simulink library "MCI_lib"  (Simulink 7.5)
settings: Solver=ode45  StartTime=0.0  StopTime=10.0  RelTol=1e-3
values from neighbouring files (symbols this model uses):
  pMCI_bool_MotCtrlTqLimEna_C = Simulink.Parameter    [MCI_par.m]
  pMCI_m_TireDiam_C = Simulink.Parameter    [MCI_par.m]
  pMCI_Nm_DrvTqLim_C = Simulink.Parameter    [MCI_par.m]
  pMCI_Nm_RcpTqLim_C = Simulink.Parameter    [MCI_par.m]
  pMCI_ratio_DrvEff_MAP = Simulink.Parameter    [MCI_par.m]
  pMCI_ratio_KmPerHrToMtrPerSec_C = Simulink.Parameter    [MCI_par.m]
  pMCI_ratio_TrsmRat_C = Simulink.Parameter    [MCI_par.m]
  pMCI_rpm_InsteadVld_C = Simulink.Parameter    [MCI_par.m]
  pMCI_s_NoOfSec_C = Simulink.Parameter    [MCI_par.m]
undefined symbols (not defined in the file or in its folder): MotCtrlWrkStsTyp, p_bool_False_M, p_bool_True_M, p_st_DrvModeFlg_C
libraries: BaseOperationLib_Browser x79, PES_CZ_FAW x6, simulink x1
(part 1 of 2)
settings Model: Creator=wuaibin  LastModifiedBy=wuaibin

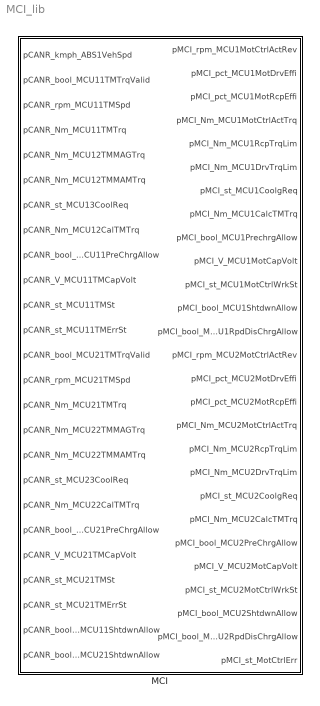
== system MCI_lib ==
  MCI : Subsystem  TreatAsAtomicUnit=on

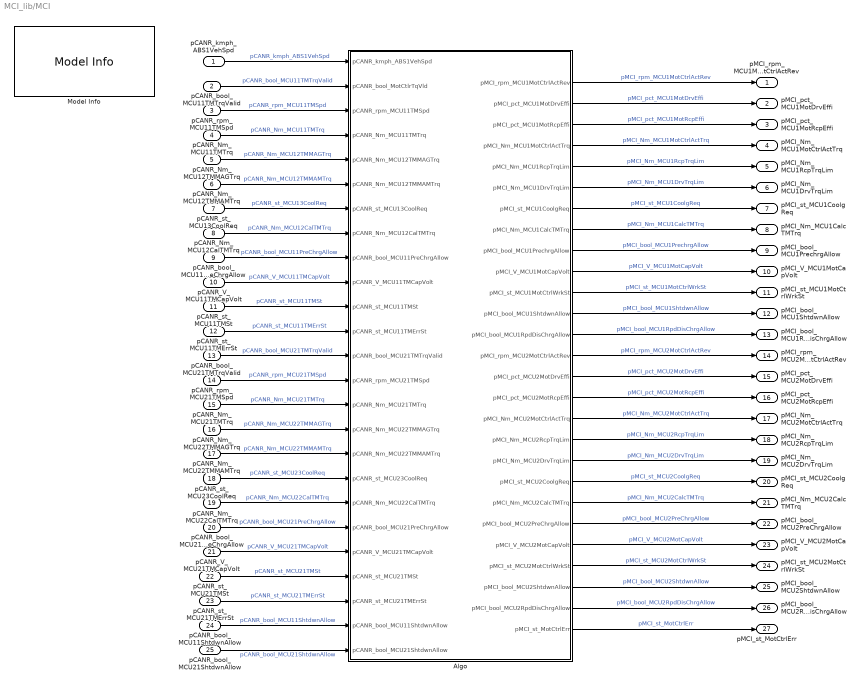
== system MCI_lib/MCI ==
  pCANR_kmph_ABS1VehSpd : Inport  OutDataType=fixdt(1, 16)  OutScaling=2^0
  pCANR_bool_MCU11TMTrqValid : Inport  Port=2
  pCANR_rpm_MCU11TMSpd : Inport  Port=3
  pCANR_Nm_MCU11TMTrq : Inport  Port=4
  pCANR_Nm_MCU12TMMAGTrq : Inport  Port=5
  pCANR_Nm_MCU12TMMAMTrq : Inport  Port=6
  pCANR_st_MCU13CoolReq : Inport  Port=7  OutDataType=fixdt(1, 16)  OutScaling=2^0
  pCANR_Nm_MCU12CalTMTrq : Inport  Port=8  OutDataType=fixdt(1, 16)  OutScaling=2^0
  pCANR_bool_MCU11PreChrgAllow : Inport  Port=9  OutDataType=fixdt(1, 16)  OutScaling=2^0
  pCANR_V_MCU11TMCapVolt : Inport  Port=10  OutDataType=fixdt(1, 16)  OutScaling=2^0
  pCANR_st_MCU11TMSt : Inport  Port=11  OutDataType=fixdt(1, 16)  OutScaling=2^0
  pCANR_st_MCU11TMErrSt : Inport  Port=12  OutDataType=fixdt(1, 16)  OutScaling=2^0
  pCANR_bool_MCU21TMTrqValid : Inport  Port=13
  pCANR_rpm_MCU21TMSpd : Inport  Port=14
  pCANR_Nm_MCU21TMTrq : Inport  Port=15
  pCANR_Nm_MCU22TMMAGTrq : Inport  Port=16  OutDataType=fixdt(1, 16)  OutScaling=2^0
  pCANR_Nm_MCU22TMMAMTrq : Inport  Port=17
  pCANR_st_MCU23CoolReq : Inport  Port=18  OutDataType=fixdt(1, 16)  OutScaling=2^0
  pCANR_Nm_MCU22CalTMTrq : Inport  Port=19  OutDataType=fixdt(1, 16)  OutScaling=2^0
  pCANR_bool_MCU21PreChrgAllow : Inport  Port=20
  pCANR_V_MCU21TMCapVolt : Inport  Port=21
  pCANR_st_MCU21TMSt : Inport  Port=22  OutDataType=fixdt(1, 16)  OutScaling=2^0
  pCANR_st_MCU21TMErrSt : Inport  Port=23  OutDataType=fixdt(1, 16)  OutScaling=2^0
  pCANR_bool_MCU11ShtdwnAllow : Inport  Port=24  OutDataType=fixdt(1, 16)  OutScaling=2^0
  pCANR_bool_MCU21ShtdwnAllow : Inport  Port=25  OutDataType=fixdt(1, 16)  OutScaling=2^0
  Algo : Subsystem
  Model Info : simulink/Model-Wide Utilities/Model Info  SystemSampleTime=-1  InitialBlockCM=None  BlockCM=None  Frame=on  DisplayStringWithTags=Model Info\nCreated: %<Created>\nCreator: wuaibin  HorizontalTextAlignment=Center  LeftAlignmentValue=0.5  SourceBlockDiagram=HQEV_HCU  TagMaxNumber=20
  pMCI_rpm_MCU1MotCtrlActRev : Outport  OutDataType=fixdt(1, 16)  OutScaling=2^0
  pMCI_pct_MCU1MotDrvEffi : Outport  Port=2  OutDataType=fixdt(1, 16)  OutScaling=2^0
  pMCI_pct_MCU1MotRcpEffi : Outport  Port=3  OutDataType=fixdt(1, 16)  OutScaling=2^0
  pMCI_Nm_MCU1MotCtrlActTrq : Outport  Port=4  OutDataType=fixdt(1, 16)  OutScaling=2^0
  pMCI_Nm_MCU1RcpTrqLim : Outport  Port=5  OutDataType=fixdt(1, 16)  OutScaling=2^0
  pMCI_Nm_MCU1DrvTrqLim : Outport  Port=6  OutDataType=fixdt(1, 16)  OutScaling=2^0
  pMCI_st_MCU1CoolgReq : Outport  Port=7  OutDataType=fixdt(1, 16)  OutScaling=2^0
  pMCI_Nm_MCU1CalcTMTrq : Outport  Port=8  OutDataType=fixdt(1, 16)  OutScaling=2^0
  pMCI_bool_MCU1PrechrgAllow : Outport  Port=9  OutDataType=fixdt(1, 16)  OutScaling=2^0
  pMCI_V_MCU1MotCapVolt : Outport  Port=10  OutDataType=fixdt(1, 16)  OutScaling=2^0
  pMCI_st_MCU1MotCtrlWrkSt : Outport  Port=11  OutDataType=fixdt(1, 16)  OutScaling=2^0
  pMCI_bool_MCU1ShtdwnAllow : Outport  Port=12  OutDataType=fixdt(1, 16)  OutScaling=2^0
  pMCI_bool_MCU1RpdDisChrgAllow : Outport  Port=13  OutDataType=fixdt(1, 16)  OutScaling=2^0
  pMCI_rpm_MCU2MotCtrlActRev : Outport  Port=14  OutDataType=fixdt(1, 16)  OutScaling=2^0
  pMCI_pct_MCU2MotDrvEffi : Outport  Port=15  OutDataType=fixdt(1, 16)  OutScaling=2^0
  pMCI_pct_MCU2MotRcpEffi : Outport  Port=16  OutDataType=fixdt(1, 16)  OutScaling=2^0
  pMCI_Nm_MCU2MotCtrlActTrq : Outport  Port=17  OutDataType=fixdt(1, 16)  OutScaling=2^0
  pMCI_Nm_MCU2RcpTrqLim : Outport  Port=18  OutDataType=fixdt(1, 16)  OutScaling=2^0
  pMCI_Nm_MCU2DrvTrqLim : Outport  Port=19  OutDataType=fixdt(1, 16)  OutScaling=2^0
  pMCI_st_MCU2CoolgReq : Outport  Port=20  OutDataType=fixdt(1, 16)  OutScaling=2^0
  pMCI_Nm_MCU2CalcTMTrq : Outport  Port=21  OutDataType=fixdt(1, 16)  OutScaling=2^0
  pMCI_bool_MCU2PreChrgAllow : Outport  Port=22  OutDataType=fixdt(1, 16)  OutScaling=2^0
  pMCI_V_MCU2MotCapVolt : Outport  Port=23  OutDataType=fixdt(1, 16)  OutScaling=2^0
  pMCI_st_MCU2MotCtrlWrkSt : Outport  Port=24  OutDataType=fixdt(1, 16)  OutScaling=2^0
  pMCI_bool_MCU2ShtdwnAllow : Outport  Port=25  OutDataType=fixdt(1, 16)  OutScaling=2^0
  pMCI_bool_MCU2RpdDisChrgAllow : Outport  Port=26  OutDataType=fixdt(1, 16)  OutScaling=2^0
  pMCI_st_MotCtrlErr : Outport  Port=27
  wires:
  pCANR_bool_MCU21TMTrqValid/1 -> Algo/13(pCANR_bool_MCU21TMTrqValid)  "pCANR_bool_MCU21TMTrqValid"
  pCANR_bool_MCU11TMTrqValid/1 -> Algo/2(pCANR_bool_MotCtlrTqVld)  "pCANR_bool_MCU11TMTrqValid"
  Algo/26(pMCI_bool_MCU2RpdDisChrgAllow) -> pMCI_bool_MCU2RpdDisChrgAllow/1  "pMCI_bool_MCU2RpdDisChrgAllow"
  Algo/13(pMCI_bool_MCU1RpdDisChrgAllow) -> pMCI_bool_MCU1RpdDisChrgAllow/1  "pMCI_bool_MCU1RpdDisChrgAllow"
  pCANR_st_MCU11TMErrSt/1 -> Algo/12(pCANR_st_MCU11TMErrSt)  "pCANR_st_MCU11TMErrSt"
  pCANR_st_MCU21TMErrSt/1 -> Algo/23(pCANR_st_MCU21TMErrSt)  "pCANR_st_MCU21TMErrSt"
  Algo/25(pMCI_bool_MCU2ShtdwnAllow) -> pMCI_bool_MCU2ShtdwnAllow/1  "pMCI_bool_MCU2ShtdwnAllow"
  Algo/12(pMCI_bool_MCU1ShtdwnAllow) -> pMCI_bool_MCU1ShtdwnAllow/1  "pMCI_bool_MCU1ShtdwnAllow"
  Algo/27(pMCI_st_MotCtrlErr) -> pMCI_st_MotCtrlErr/1  "pMCI_st_MotCtrlErr"
  pCANR_st_MCU21TMSt/1 -> Algo/22(pCANR_st_MCU21TMSt)  "pCANR_st_MCU21TMSt"
  pCANR_V_MCU21TMCapVolt/1 -> Algo/21(pCANR_V_MCU21TMCapVolt)  "pCANR_V_MCU21TMCapVolt"
  pCANR_bool_MCU21PreChrgAllow/1 -> Algo/20(pCANR_bool_MCU21PreChrgAllow)  "pCANR_bool_MCU21PreChrgAllow"
  pCANR_Nm_MCU22CalTMTrq/1 -> Algo/19(pCANR_Nm_MCU22CalTMTrq)  "pCANR_Nm_MCU22CalTMTrq"
  pCANR_st_MCU23CoolReq/1 -> Algo/18(pCANR_st_MCU23CoolReq)  "pCANR_st_MCU23CoolReq"
  pCANR_Nm_MCU22TMMAMTrq/1 -> Algo/17(pCANR_Nm_MCU22TMMAMTrq)  "pCANR_Nm_MCU22TMMAMTrq"
  pCANR_Nm_MCU22TMMAGTrq/1 -> Algo/16(pCANR_Nm_MCU22TMMAGTrq)  "pCANR_Nm_MCU22TMMAGTrq"
  pCANR_Nm_MCU21TMTrq/1 -> Algo/15(pCANR_Nm_MCU21TMTrq)  "pCANR_Nm_MCU21TMTrq"
  pCANR_rpm_MCU21TMSpd/1 -> Algo/14(pCANR_rpm_MCU21TMSpd)  "pCANR_rpm_MCU21TMSpd"
  Algo/1(pMCI_rpm_MCU1MotCtrlActRev) -> pMCI_rpm_MCU1MotCtrlActRev/1  "pMCI_rpm_MCU1MotCtrlActRev"
  pCANR_kmph_ABS1VehSpd/1 -> Algo/1(pCANR_kmph_ABS1VehSpd)  "pCANR_kmph_ABS1VehSpd"
  Algo/2(pMCI_pct_MCU1MotDrvEffi) -> pMCI_pct_MCU1MotDrvEffi/1  "pMCI_pct_MCU1MotDrvEffi"
  pCANR_rpm_MCU11TMSpd/1 -> Algo/3(pCANR_rpm_MCU11TMSpd)  "pCANR_rpm_MCU11TMSpd"
  Algo/3(pMCI_pct_MCU1MotRcpEffi) -> pMCI_pct_MCU1MotRcpEffi/1  "pMCI_pct_MCU1MotRcpEffi"
  pCANR_Nm_MCU11TMTrq/1 -> Algo/4(pCANR_Nm_MCU11TMTrq)  "pCANR_Nm_MCU11TMTrq"
  Algo/4(pMCI_Nm_MCU1MotCtrlActTrq) -> pMCI_Nm_MCU1MotCtrlActTrq/1  "pMCI_Nm_MCU1MotCtrlActTrq"
  pCANR_Nm_MCU12TMMAGTrq/1 -> Algo/5(pCANR_Nm_MCU12TMMAGTrq)  "pCANR_Nm_MCU12TMMAGTrq"
  Algo/5(pMCI_Nm_MCU1RcpTrqLim) -> pMCI_Nm_MCU1RcpTrqLim/1  "pMCI_Nm_MCU1RcpTrqLim"
  Algo/6(pMCI_Nm_MCU1DrvTrqLim) -> pMCI_Nm_MCU1DrvTrqLim/1  "pMCI_Nm_MCU1DrvTrqLim"
  pCANR_Nm_MCU12TMMAMTrq/1 -> Algo/6(pCANR_Nm_MCU12TMMAMTrq)  "pCANR_Nm_MCU12TMMAMTrq"
  Algo/7(pMCI_st_MCU1CoolgReq) -> pMCI_st_MCU1CoolgReq/1  "pMCI_st_MCU1CoolgReq"
  pCANR_st_MCU13CoolReq/1 -> Algo/7(pCANR_st_MCU13CoolReq)  "pCANR_st_MCU13CoolReq"
  Algo/8(pMCI_Nm_MCU1CalcTMTrq) -> pMCI_Nm_MCU1CalcTMTrq/1  "pMCI_Nm_MCU1CalcTMTrq"
  pCANR_Nm_MCU12CalTMTrq/1 -> Algo/8(pCANR_Nm_MCU12CalTMTrq)  "pCANR_Nm_MCU12CalTMTrq"
  pCANR_bool_MCU11PreChrgAllow/1 -> Algo/9(pCANR_bool_MCU11PreChrgAllow)  "pCANR_bool_MCU11PreChrgAllow"
  Algo/9(pMCI_bool_MCU1PrechrgAllow) -> pMCI_bool_MCU1PrechrgAllow/1  "pMCI_bool_MCU1PrechrgAllow"
  pCANR_V_MCU11TMCapVolt/1 -> Algo/10(pCANR_V_MCU11TMCapVolt)  "pCANR_V_MCU11TMCapVolt"
  pCANR_st_MCU11TMSt/1 -> Algo/11(pCANR_st_MCU11TMSt)  "pCANR_st_MCU11TMSt"
  Algo/10(pMCI_V_MCU1MotCapVolt) -> pMCI_V_MCU1MotCapVolt/1  "pMCI_V_MCU1MotCapVolt"
  Algo/11(pMCI_st_MCU1MotCtrlWrkSt) -> pMCI_st_MCU1MotCtrlWrkSt/1  "pMCI_st_MCU1MotCtrlWrkSt"
  Algo/14(pMCI_rpm_MCU2MotCtrlActRev) -> pMCI_rpm_MCU2MotCtrlActRev/1  "pMCI_rpm_MCU2MotCtrlActRev"
  Algo/15(pMCI_pct_MCU2MotDrvEffi) -> pMCI_pct_MCU2MotDrvEffi/1  "pMCI_pct_MCU2MotDrvEffi"
  Algo/16(pMCI_pct_MCU2MotRcpEffi) -> pMCI_pct_MCU2MotRcpEffi/1  "pMCI_pct_MCU2MotRcpEffi"
  Algo/17(pMCI_Nm_MCU2MotCtrlActTrq) -> pMCI_Nm_MCU2MotCtrlActTrq/1  "pMCI_Nm_MCU2MotCtrlActTrq"
  Algo/18(pMCI_Nm_MCU2RcpTrqLim) -> pMCI_Nm_MCU2RcpTrqLim/1  "pMCI_Nm_MCU2RcpTrqLim"
  Algo/19(pMCI_Nm_MCU2DrvTrqLim) -> pMCI_Nm_MCU2DrvTrqLim/1  "pMCI_Nm_MCU2DrvTrqLim"
  Algo/20(pMCI_st_MCU2CoolgReq) -> pMCI_st_MCU2CoolgReq/1  "pMCI_st_MCU2CoolgReq"
  Algo/21(pMCI_Nm_MCU2CalcTMTrq) -> pMCI_Nm_MCU2CalcTMTrq/1  "pMCI_Nm_MCU2CalcTMTrq"
  Algo/22(pMCI_bool_MCU2PreChrgAllow) -> pMCI_bool_MCU2PreChrgAllow/1  "pMCI_bool_MCU2PreChrgAllow"
  Algo/23(pMCI_V_MCU2MotCapVolt) -> pMCI_V_MCU2MotCapVolt/1  "pMCI_V_MCU2MotCapVolt"
  Algo/24(pMCI_st_MCU2MotCtrlWrkSt) -> pMCI_st_MCU2MotCtrlWrkSt/1  "pMCI_st_MCU2MotCtrlWrkSt"
  pCANR_bool_MCU11ShtdwnAllow/1 -> Algo/24(pCANR_bool_MCU11ShtdwnAllow)  "pCANR_bool_MCU11ShtdwnAllow"
  pCANR_bool_MCU21ShtdwnAllow/1 -> Algo/25(pCANR_bool_MCU21ShtdwnAllow)  "pCANR_bool_MCU21ShtdwnAllow"

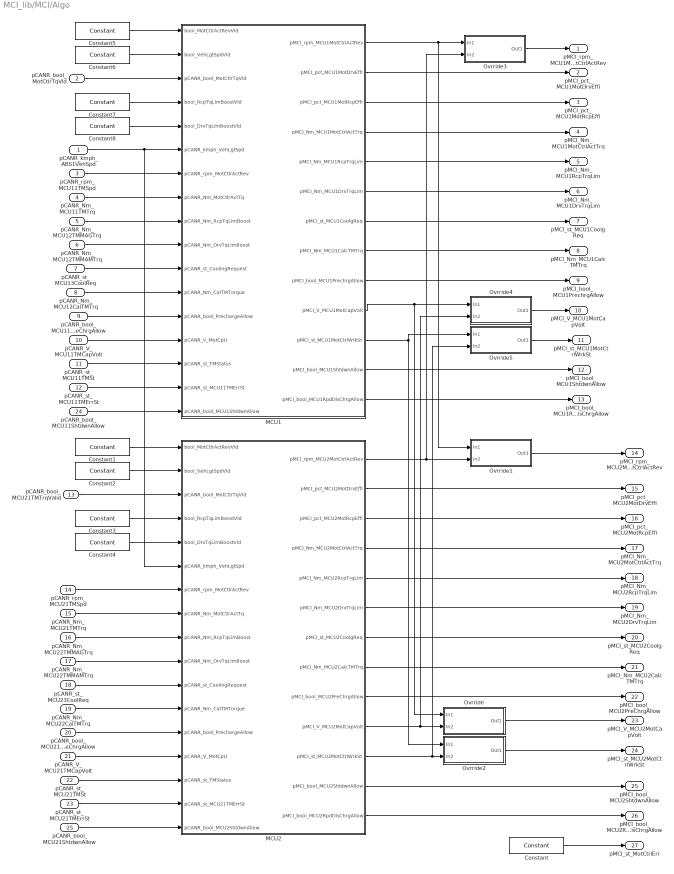
== system MCI_lib/MCI/Algo ==
  pCANR_kmph_ABS1VehSpd : Inport  OutDataType=fixdt(1, 16)  OutScaling=2^0
  pCANR_bool_MotCtlrTqVld : Inport  Port=2
  pCANR_rpm_MCU11TMSpd : Inport  Port=3
  pCANR_Nm_MCU11TMTrq : Inport  Port=4
  pCANR_Nm_MCU12TMMAGTrq : Inport  Port=5
  pCANR_Nm_MCU12TMMAMTrq : Inport  Port=6
  pCANR_st_MCU13CoolReq : Inport  Port=7  OutDataType=fixdt(1, 16)  OutScaling=2^0
  pCANR_Nm_MCU12CalTMTrq : Inport  Port=8  OutDataType=fixdt(1, 16)  OutScaling=2^0
  pCANR_bool_MCU11PreChrgAllow : Inport  Port=9  OutDataType=fixdt(1, 16)  OutScaling=2^0
  pCANR_V_MCU11TMCapVolt : Inport  Port=10  OutDataType=fixdt(1, 16)  OutScaling=2^0
  pCANR_st_MCU11TMSt : Inport  Port=11  OutDataType=fixdt(1, 16)  OutScaling=2^0
  pCANR_st_MCU11TMErrSt : Inport  Port=12  OutDataType=fixdt(1, 16)  OutScaling=2^0
  pCANR_bool_MCU21TMTrqValid : Inport  Port=13
  pCANR_rpm_MCU21TMSpd : Inport  Port=14
  pCANR_Nm_MCU21TMTrq : Inport  Port=15
  pCANR_Nm_MCU22TMMAGTrq : Inport  Port=16  OutDataType=fixdt(1, 16)  OutScaling=2^0
  pCANR_Nm_MCU22TMMAMTrq : Inport  Port=17
  pCANR_st_MCU23CoolReq : Inport  Port=18  OutDataType=fixdt(1, 16)  OutScaling=2^0
  pCANR_Nm_MCU22CalTMTrq : Inport  Port=19  OutDataType=fixdt(1, 16)  OutScaling=2^0
  pCANR_bool_MCU21PreChrgAllow : Inport  Port=20
  pCANR_V_MCU21TMCapVolt : Inport  Port=21
  pCANR_st_MCU21TMSt : Inport  Port=22  OutDataType=fixdt(1, 16)  OutScaling=2^0
  pCANR_st_MCU21TMErrSt : Inport  Port=23  OutDataType=fixdt(1, 16)  OutScaling=2^0
  pCANR_bool_MCU11ShtdwnAllow : Inport  Port=24  OutDataType=fixdt(1, 16)  OutScaling=2^0
  pCANR_bool_MCU21ShtdwnAllow : Inport  Port=25  OutDataType=fixdt(1, 16)  OutScaling=2^0
  Constant : BaseOperationLib_Browser/Sources&Sinks/Constant  Value=0  OutMin=[]  OutMax=[]  OutDataTypeMode=uint32  OutDataType=fixdt(1, 16)  ConRadixGroup=Use specified scaling  OutScaling=2^0  OutDataTypeStr=uint32
  Constant{1,3..5,7..8} (6 alike) : BaseOperationLib_Browser/Sources&Sinks/Constant  Value=p_bool_True_M  OutMin=[]  OutMax=[]  OutDataTypeMode=uint32  OutDataType=fixdt(1, 16)  ConRadixGroup=Use specified scaling  OutScaling=2^0  OutDataTypeStr=uint32
  Constant2 : BaseOperationLib_Browser/Sources&Sinks/Constant  Value=p_bool_False_M  OutMin=[]  OutMax=[]  OutDataTypeMode=uint32  OutDataType=fixdt(1, 16)  ConRadixGroup=Use specified scaling  OutScaling=2^0  OutDataTypeStr=uint32
  Constant6 : BaseOperationLib_Browser/Sources&Sinks/Constant  Value=p_bool_False_M  OutMin=[]  OutMax=[]  OutDataTypeMode=uint32  OutDataType=fixdt(1, 16)  ConRadixGroup=Use specified scaling  OutScaling=2^0  OutDataTypeStr=uint32
  MCU1 : Subsystem
  MCU2 : Subsystem
  Ovrride : Subsystem
  Ovrride1 : Subsystem
  Ovrride2 : Subsystem
  Ovrride3 : Subsystem
  Ovrride4 : Subsystem
  Ovrride5 : Subsystem
  pMCI_rpm_MCU1MotCtrlActRev : Outport  OutDataType=fixdt(1, 16)  OutScaling=2^0
  pMCI_pct_MCU1MotDrvEffi : Outport  Port=2  OutDataType=fixdt(1, 16)  OutScaling=2^0
  pMCI_pct_MCU1MotRcpEffi : Outport  Port=3  OutDataType=fixdt(1, 16)  OutScaling=2^0
  pMCI_Nm_MCU1MotCtrlActTrq : Outport  Port=4  OutDataType=fixdt(1, 16)  OutScaling=2^0
  pMCI_Nm_MCU1RcpTrqLim : Outport  Port=5  OutDataType=fixdt(1, 16)  OutScaling=2^0
  pMCI_Nm_MCU1DrvTrqLim : Outport  Port=6  OutDataType=fixdt(1, 16)  OutScaling=2^0
  pMCI_st_MCU1CoolgReq : Outport  Port=7  OutDataType=fixdt(1, 16)  OutScaling=2^0
  pMCI_Nm_MCU1CalcTMTrq : Outport  Port=8  OutDataType=fixdt(1, 16)  OutScaling=2^0
  pMCI_bool_MCU1PrechrgAllow : Outport  Port=9  OutDataType=fixdt(1, 16)  OutScaling=2^0
  pMCI_V_MCU1MotCapVolt : Outport  Port=10  OutDataType=fixdt(1, 16)  OutScaling=2^0
  pMCI_st_MCU1MotCtrlWrkSt : Outport  Port=11  OutDataType=fixdt(1, 16)  OutScaling=2^0
  pMCI_bool_MCU1ShtdwnAllow : Outport  Port=12  OutDataType=fixdt(1, 16)  OutScaling=2^0
  pMCI_bool_MCU1RpdDisChrgAllow : Outport  Port=13  OutDataType=fixdt(1, 16)  OutScaling=2^0
  pMCI_rpm_MCU2MotCtrlActRev : Outport  Port=14  OutDataType=fixdt(1, 16)  OutScaling=2^0
  pMCI_pct_MCU2MotDrvEffi : Outport  Port=15  OutDataType=fixdt(1, 16)  OutScaling=2^0
  pMCI_pct_MCU2MotRcpEffi : Outport  Port=16  OutDataType=fixdt(1, 16)  OutScaling=2^0
  pMCI_Nm_MCU2MotCtrlActTrq : Outport  Port=17  OutDataType=fixdt(1, 16)  OutScaling=2^0
  pMCI_Nm_MCU2RcpTrqLim : Outport  Port=18  OutDataType=fixdt(1, 16)  OutScaling=2^0
  pMCI_Nm_MCU2DrvTrqLim : Outport  Port=19  OutDataType=fixdt(1, 16)  OutScaling=2^0
  pMCI_st_MCU2CoolgReq : Outport  Port=20  OutDataType=fixdt(1, 16)  OutScaling=2^0
  pMCI_Nm_MCU2CalcTMTrq : Outport  Port=21  OutDataType=fixdt(1, 16)  OutScaling=2^0
  pMCI_bool_MCU2PreChrgAllow : Outport  Port=22  OutDataType=fixdt(1, 16)  OutScaling=2^0
  pMCI_V_MCU2MotCapVolt : Outport  Port=23  OutDataType=fixdt(1, 16)  OutScaling=2^0
  pMCI_st_MCU2MotCtrlWrkSt : Outport  Port=24  OutDataType=fixdt(1, 16)  OutScaling=2^0
  pMCI_bool_MCU2ShtdwnAllow : Outport  Port=25  OutDataType=fixdt(1, 16)  OutScaling=2^0
  pMCI_bool_MCU2RpdDisChrgAllow : Outport  Port=26  OutDataType=fixdt(1, 16)  OutScaling=2^0
  pMCI_st_MotCtrlErr : Outport  Port=27  OutDataType=fixdt(1, 16)  OutScaling=2^0
  wires:
  Constant8/1 -> MCU1/5(bool_DrvTqLimBoostVld)
  Constant7/1 -> MCU1/4(bool_RcpTqLimBoostVld)
  Constant6/1 -> MCU1/2(bool_VehLgtSpdVld)
  Constant5/1 -> MCU1/1(bool_MotCtlrActRevVld)
  Constant4/1 -> MCU2/5(bool_DrvTqLimBoostVld)
  Constant3/1 -> MCU2/4(bool_RcpTqLimBoostVld)
  Constant2/1 -> MCU2/2(bool_VehLgtSpdVld)
  Constant1/1 -> MCU2/1(bool_MotCtlrActRevVld)
  pCANR_bool_MCU21TMTrqValid/1 -> MCU2/3(pCANR_bool_MotCtlrTqVld)
  Constant/1 -> pMCI_st_MotCtrlErr/1
  pCANR_st_MCU11TMErrSt/1 -> MCU1/16(pCANR_st_MCU11TMErrSt)
  MCU2/13(pMCI_bool_MCU2RpdDisChrgAllow) -> pMCI_bool_MCU2RpdDisChrgAllow/1
  MCU1/13(pMCI_bool_MCU1RpdDisChrgAllow) -> pMCI_bool_MCU1RpdDisChrgAllow/1
  MCU2/1(pMCI_rpm_MCU2MotCtrlActRev) -> Ovrride1/2(In2), Ovrride3/2(In2)
  pCANR_st_MCU21TMErrSt/1 -> MCU2/16(pCANR_st_MCU21TMErrSt)
  MCU1/1(pMCI_rpm_MCU1MotCtrlActRev) -> Ovrride1/1(In1), Ovrride3/1(In1)
  MCU1/9(pMCI_bool_MCU1PrechrgAllow) -> pMCI_bool_MCU1PrechrgAllow/1
  Ovrride/1(Out1) -> pMCI_V_MCU2MotCapVolt/1
  Ovrride2/1(Out1) -> pMCI_st_MCU2MotCtrlWrkSt/1
  Ovrride1/1(Out1) -> pMCI_rpm_MCU2MotCtrlActRev/1
  MCU2/9(pMCI_bool_MCU2PreChrgAllow) -> pMCI_bool_MCU2PreChrgAllow/1
  MCU2/11(pMCI_st_MCU2MotCtrlWrkSt) -> Ovrride2/2(In2), Ovrride5/2(In2)
  MCU2/10(pMCI_V_MCU2MotCapVolt) -> Ovrride/2(In2), Ovrride4/2(In2)
  MCU2/12(pMCI_bool_MCU2ShtdwnAllow) -> pMCI_bool_MCU2ShtdwnAllow/1
  MCU1/12(pMCI_bool_MCU1ShtdwnAllow) -> pMCI_bool_MCU1ShtdwnAllow/1
  MCU1/11(pMCI_st_MCU1MotCtrlWrkSt) -> Ovrride2/1(In1), Ovrride5/1(In1)
  MCU1/8(pMCI_Nm_MCU1CalcTMTrq) -> pMCI_Nm_MCU1CalcTMTrq/1
  MCU1/7(pMCI_st_MCU1CoolgReq) -> pMCI_st_MCU1CoolgReq/1
  MCU1/6(pMCI_Nm_MCU1DrvTrqLim) -> pMCI_Nm_MCU1DrvTrqLim/1
  MCU2/8(pMCI_Nm_MCU2CalcTMTrq) -> pMCI_Nm_MCU2CalcTMTrq/1
  MCU2/7(pMCI_st_MCU2CoolgReq) -> pMCI_st_MCU2CoolgReq/1
  MCU1/10(pMCI_V_MCU1MotCapVolt) -> Ovrride/1(In1), Ovrride4/1(In1)
  pCANR_st_MCU21TMSt/1 -> MCU2/15(pCANR_st_TMStatus)
  pCANR_rpm_MCU21TMSpd/1 -> MCU2/7(pCANR_rpm_MotCtlrActRev)
  pCANR_Nm_MCU21TMTrq/1 -> MCU2/8(pCANR_Nm_MotCtlrActTq)
  pCANR_Nm_MCU22TMMAGTrq/1 -> MCU2/9(pCANR_Nm_RcpTqLimBoost)
  pCANR_Nm_MCU22TMMAMTrq/1 -> MCU2/10(pCANR_Nm_DrvTqLimBoost)
  pCANR_st_MCU23CoolReq/1 -> MCU2/11(pCANR_st_CoolingRequest)
  pCANR_Nm_MCU22CalTMTrq/1 -> MCU2/12(pCANR_Nm_CalTMTorque)
  pCANR_bool_MCU21PreChrgAllow/1 -> MCU2/13(pCANR_bool_PrechargeAllow)
  pCANR_V_MCU21TMCapVolt/1 -> MCU2/14(pCANR_V_MotCpU)
  MCU2/6(pMCI_Nm_MCU2DrvTrqLim) -> pMCI_Nm_MCU2DrvTrqLim/1
  MCU2/5(pMCI_Nm_MCU2RcpTrqLim) -> pMCI_Nm_MCU2RcpTrqLim/1
  MCU2/4(pMCI_Nm_MCU2MotCtrlActTrq) -> pMCI_Nm_MCU2MotCtrlActTrq/1
  MCU2/3(pMCI_pct_MCU2MotRcpEffi) -> pMCI_pct_MCU2MotRcpEffi/1
  MCU2/2(pMCI_pct_MCU2MotDrvEffi) -> pMCI_pct_MCU2MotDrvEffi/1
  pCANR_st_MCU11TMSt/1 -> MCU1/15(pCANR_st_TMStatus)
  pCANR_st_MCU13CoolReq/1 -> MCU1/11(pCANR_st_CoolingRequest)
  pCANR_Nm_MCU12CalTMTrq/1 -> MCU1/12(pCANR_Nm_CalTMTorque)
  pCANR_kmph_ABS1VehSpd/1 -> MCU2/6(pCANR_kmph_VehLgtSpd), MCU1/6(pCANR_kmph_VehLgtSpd)
  pCANR_V_MCU11TMCapVolt/1 -> MCU1/14(pCANR_V_MotCpU)
  pCANR_bool_MCU11PreChrgAllow/1 -> MCU1/13(pCANR_bool_PrechargeAllow)
  pCANR_rpm_MCU11TMSpd/1 -> MCU1/7(pCANR_rpm_MotCtlrActRev)
  MCU1/5(pMCI_Nm_MCU1RcpTrqLim) -> pMCI_Nm_MCU1RcpTrqLim/1
  MCU1/4(pMCI_Nm_MCU1MotCtrlActTrq) -> pMCI_Nm_MCU1MotCtrlActTrq/1
  MCU1/3(pMCI_pct_MCU1MotRcpEffi) -> pMCI_pct_MCU1MotRcpEffi/1
  MCU1/2(pMCI_pct_MCU1MotDrvEffi) -> pMCI_pct_MCU1MotDrvEffi/1
  pCANR_Nm_MCU12TMMAMTrq/1 -> MCU1/10(pCANR_Nm_DrvTqLimBoost)
  pCANR_Nm_MCU12TMMAGTrq/1 -> MCU1/9(pCANR_Nm_RcpTqLimBoost)
  pCANR_bool_MotCtlrTqVld/1 -> MCU1/3(pCANR_bool_MotCtlrTqVld)
  pCANR_Nm_MCU11TMTrq/1 -> MCU1/8(pCANR_Nm_MotCtlrActTq)
  Ovrride3/1(Out1) -> pMCI_rpm_MCU1MotCtrlActRev/1
  Ovrride4/1(Out1) -> pMCI_V_MCU1MotCapVolt/1
  Ovrride5/1(Out1) -> pMCI_st_MCU1MotCtrlWrkSt/1
  pCANR_bool_MCU11ShtdwnAllow/1 -> MCU1/17(pCANR_bool_MCU1ShtdwnAllow)
  pCANR_bool_MCU21ShtdwnAllow/1 -> MCU2/17(pCANR_bool_MCU2ShtdwnAllow)

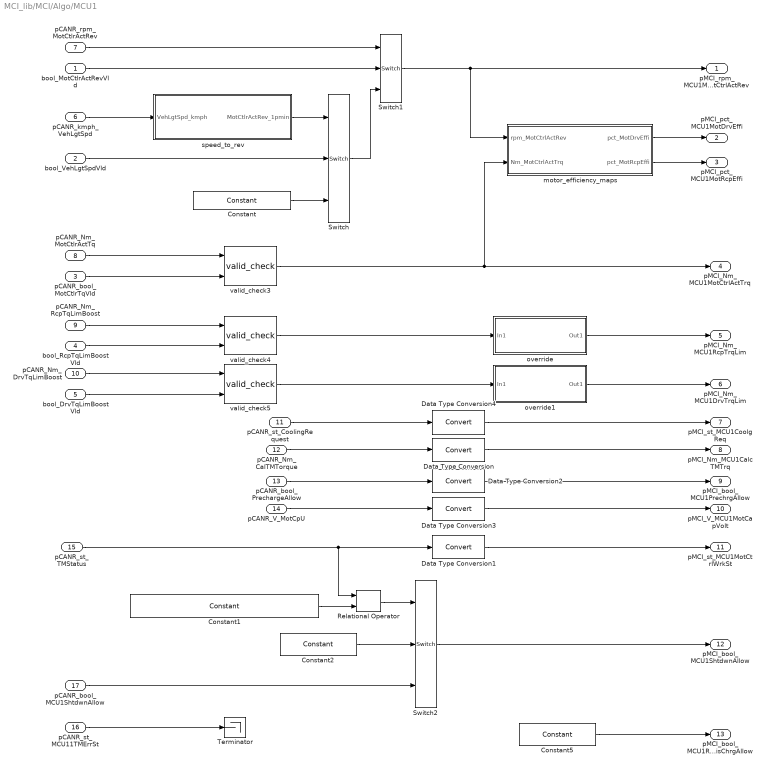
== system MCI_lib/MCI/Algo/MCU1 ==
  bool_MotCtlrActRevVld : Inport  OutDataType=fixdt(1, 16)  OutScaling=2^0
  bool_VehLgtSpdVld : Inport  Port=2  OutDataType=fixdt(1, 16)  OutScaling=2^0
  pCANR_bool_MotCtlrTqVld : Inport  Port=3  OutDataType=fixdt(1, 16)  OutScaling=2^0
  bool_RcpTqLimBoostVld : Inport  Port=4  OutDataType=fixdt(1, 16)  OutScaling=2^0
  bool_DrvTqLimBoostVld : Inport  Port=5  OutDataType=fixdt(1, 16)  OutScaling=2^0
  pCANR_kmph_VehLgtSpd : Inport  Port=6  OutDataType=fixdt(1, 16)  OutScaling=2^0
  pCANR_rpm_MotCtlrActRev : Inport  Port=7  OutDataType=fixdt(1, 16)  OutScaling=2^0
  pCANR_Nm_MotCtlrActTq : Inport  Port=8  OutDataType=fixdt(1, 16)  OutScaling=2^0
  pCANR_Nm_RcpTqLimBoost : Inport  Port=9  OutDataType=fixdt(1, 16)  OutScaling=2^0
  pCANR_Nm_DrvTqLimBoost : Inport  Port=10  OutDataType=fixdt(1, 16)  OutScaling=2^0
  pCANR_st_CoolingRequest : Inport  Port=11  OutDataType=fixdt(1, 16)  OutScaling=2^0
  pCANR_Nm_CalTMTorque : Inport  Port=12  OutDataType=fixdt(1, 16)  OutScaling=2^0
  pCANR_bool_PrechargeAllow : Inport  Port=13  OutDataType=fixdt(1, 16)  OutScaling=2^0
  pCANR_V_MotCpU : Inport  Port=14  OutDataType=fixdt(1, 16)  OutScaling=2^0
  pCANR_st_TMStatus : Inport  Port=15  OutDataType=fixdt(1, 16)  OutScaling=2^0
  pCANR_st_MCU11TMErrSt : Inport  Port=16  OutDataType=fixdt(1, 16)  OutScaling=2^0
  pCANR_bool_MCU1ShtdwnAllow : Inport  Port=17  OutDataType=fixdt(1, 16)  OutScaling=2^0
  Constant : BaseOperationLib_Browser/Sources&Sinks/Constant  Value=pMCI_rpm_InsteadVld_C  OutMin=[]  OutMax=[]  OutDataTypeMode=single  OutDataType=fixdt(1, 16)  ConRadixGroup=Use specified scaling  OutScaling=2^0  OutDataTypeStr=single
  Constant1 : BaseOperationLib_Browser/Sources&Sinks/Constant  Value=uint8(MotCtrlWrkStsTyp.MCWS_TORQUE_CONTROL)  OutMin=[]  OutMax=[]  OutDataType=fixdt(1, 16)  ConRadixGroup=Use specified scaling  OutScaling=2^0  OutDataTypeStr=Inherit: Inherit from 'Constant value'
  Constant2 : BaseOperationLib_Browser/Sources&Sinks/Constant  Value=p_bool_False_M  OutMin=[]  OutMax=[]  OutDataType=fixdt(1, 16)  ConRadixGroup=Use specified scaling  OutScaling=2^0  OutDataTypeStr=Inherit: Inherit from 'Constant value'
  Constant5 : BaseOperationLib_Browser/Sources&Sinks/Constant  Value=p_bool_True_M  OutMin=[]  OutMax=[]  OutDataType=fixdt(1, 16)  ConRadixGroup=Use specified scaling  OutScaling=2^0  OutDataTypeStr=Inherit: Inherit from 'Constant value'
  Data Type Conversion{,1..4} (5 alike) : DataTypeConversion  OutDataType=fixdt(1, 16)  OutScaling=2^0
  Relational Operator : BaseOperationLib_Browser/Logic Operations Changed/Relational Operator  Operator=~=  InputSameDT=on  LogicOutDataTypeMode=Specify via dialog  LogicDataType=PDT_Bool  OutDataTypeStr=PDT_Bool
  Switch : BaseOperationLib_Browser/Signal Routing Changed/Switch  Criteria=u2 ~= 0  Threshold=1  InputSameDT=on  OutMin=[]  OutMax=[]  OutDataType=fixdt(1,16,0)  OutScaling=[]  SaturateOnIntegerOverflow=on
  Switch1 : BaseOperationLib_Browser/Signal Routing Changed/Switch  Criteria=u2 ~= 0  Threshold=1  InputSameDT=on  OutMin=[]  OutMax=[]  OutDataType=fixdt(1,16,0)  OutScaling=[]  SaturateOnIntegerOverflow=on
  Switch2 : BaseOperationLib_Browser/Signal Routing Changed/Switch  Criteria=u2 ~= 0  Threshold=1  InputSameDT=on  OutMin=[]  OutMax=[]  OutDataType=fixdt(1,16,0)  OutScaling=[]  SaturateOnIntegerOverflow=on
  Terminator : Terminator
  motor_efficiency_maps : Subsystem
  override : Subsystem
  override1 : Subsystem
  speed_to_rev : Subsystem
  valid_check3 : PES_CZ_FAW/Discontinuities/valid_check  SystemSampleTime=-1  init=0
  valid_check4 : PES_CZ_FAW/Discontinuities/valid_check  SystemSampleTime=-1  init=0
  valid_check5 : PES_CZ_FAW/Discontinuities/valid_check  SystemSampleTime=-1  init=0
  pMCI_rpm_MCU1MotCtrlActRev : Outport  OutDataType=fixdt(1, 16)  OutScaling=2^0
  pMCI_pct_MCU1MotDrvEffi : Outport  Port=2  OutDataType=fixdt(1, 16)  OutScaling=2^0
  pMCI_pct_MCU1MotRcpEffi : Outport  Port=3  OutDataType=fixdt(1, 16)  OutScaling=2^0
  pMCI_Nm_MCU1MotCtrlActTrq : Outport  Port=4  OutDataType=fixdt(1, 16)  OutScaling=2^0
  pMCI_Nm_MCU1RcpTrqLim : Outport  Port=5  OutDataType=fixdt(1, 16)  OutScaling=2^0
  pMCI_Nm_MCU1DrvTrqLim : Outport  Port=6  OutDataType=fixdt(1, 16)  OutScaling=2^0
  pMCI_st_MCU1CoolgReq : Outport  Port=7  OutDataType=fixdt(1, 16)  OutScaling=2^0
  pMCI_Nm_MCU1CalcTMTrq : Outport  Port=8  OutDataType=fixdt(1, 16)  OutScaling=2^0
  pMCI_bool_MCU1PrechrgAllow : Outport  Port=9  OutDataType=fixdt(1, 16)  OutScaling=2^0
  pMCI_V_MCU1MotCapVolt : Outport  Port=10  OutDataType=fixdt(1, 16)  OutScaling=2^0
  pMCI_st_MCU1MotCtrlWrkSt : Outport  Port=11  OutDataType=fixdt(1, 16)  OutScaling=2^0
  pMCI_bool_MCU1ShtdwnAllow : Outport  Port=12
  pMCI_bool_MCU1RpdDisChrgAllow : Outport  Port=13  OutDataType=fixdt(1, 16)  OutScaling=2^0
  wires:
  pCANR_st_MCU11TMErrSt/1 -> Terminator/1
  Constant1/1 -> Relational Operator/2
  Constant5/1 -> pMCI_bool_MCU1RpdDisChrgAllow/1
  Switch1/1 -> pMCI_rpm_MCU1MotCtrlActRev/1, motor_efficiency_maps/1(rpm_MotCtrlActRev)
  bool_VehLgtSpdVld/1 -> Switch/2
  Constant/1 -> Switch/3
  speed_to_rev/1(MotCtlrActRev_1pmin) -> Switch/1
  pCANR_kmph_VehLgtSpd/1 -> speed_to_rev/1(VehLgtSpd_kmph)
  bool_MotCtlrActRevVld/1 -> Switch1/2
  pCANR_rpm_MotCtlrActRev/1 -> Switch1/1
  Switch/1 -> Switch1/3
  motor_efficiency_maps/1(pct_MotDrvEffi) -> pMCI_pct_MCU1MotDrvEffi/1
  motor_efficiency_maps/2(pct_MotRcpEffi) -> pMCI_pct_MCU1MotRcpEffi/1
  pCANR_Nm_MotCtlrActTq/1 -> valid_check3/1
  pCANR_bool_MotCtlrTqVld/1 -> valid_check3/2
  valid_check3/1 -> motor_efficiency_maps/2(Nm_MotCtrlActTrq), pMCI_Nm_MCU1MotCtrlActTrq/1
  bool_RcpTqLimBoostVld/1 -> valid_check4/2
  bool_DrvTqLimBoostVld/1 -> valid_check5/2
  pCANR_Nm_RcpTqLimBoost/1 -> valid_check4/1
  pCANR_Nm_DrvTqLimBoost/1 -> valid_check5/1
  valid_check4/1 -> override/1(In1)
  valid_check5/1 -> override1/1(In1)
  override/1(Out1) -> pMCI_Nm_MCU1RcpTrqLim/1
  override1/1(Out1) -> pMCI_Nm_MCU1DrvTrqLim/1
  Data Type Conversion1/1 -> pMCI_st_MCU1MotCtrlWrkSt/1
  pCANR_st_TMStatus/1 -> Relational Operator/1, Data Type Conversion1/1
  pCANR_st_CoolingRequest/1 -> Data Type Conversion4/1
  pCANR_Nm_CalTMTorque/1 -> Data Type Conversion/1
  pCANR_V_MotCpU/1 -> Data Type Conversion3/1
  pCANR_bool_PrechargeAllow/1 -> Data Type Conversion2/1
  Data Type Conversion/1 -> pMCI_Nm_MCU1CalcTMTrq/1
  Data Type Conversion2/1 -> pMCI_bool_MCU1PrechrgAllow/1
  Data Type Conversion3/1 -> pMCI_V_MCU1MotCapVolt/1
  Data Type Conversion4/1 -> pMCI_st_MCU1CoolgReq/1
  Relational Operator/1 -> Switch2/1
  pCANR_bool_MCU1ShtdwnAllow/1 -> Switch2/3
  Switch2/1 -> pMCI_bool_MCU1ShtdwnAllow/1
  Constant2/1 -> Switch2/2

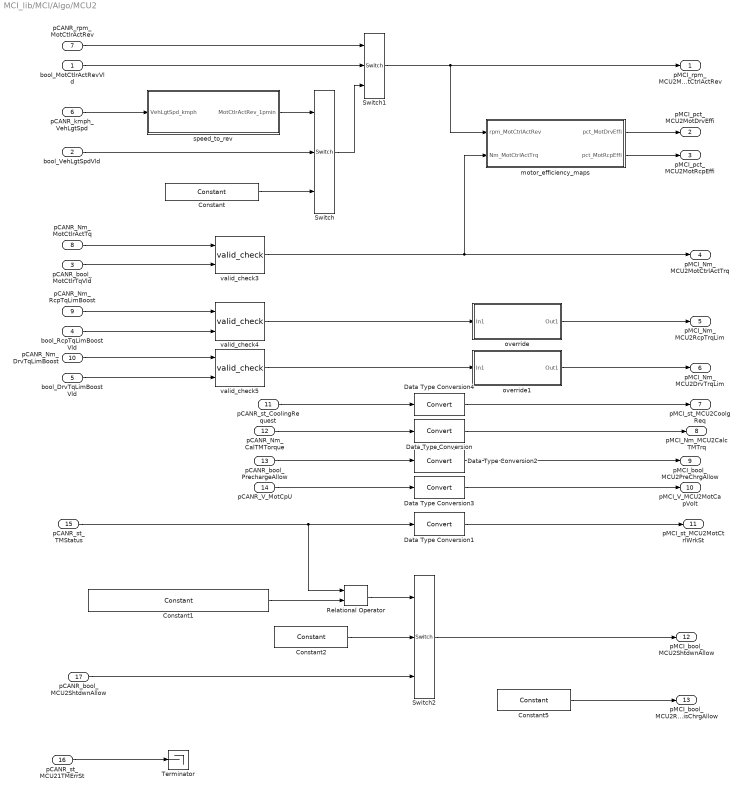
== system MCI_lib/MCI/Algo/MCU2 ==
  bool_MotCtlrActRevVld : Inport  OutDataType=fixdt(1, 16)  OutScaling=2^0
  bool_VehLgtSpdVld : Inport  Port=2  OutDataType=fixdt(1, 16)  OutScaling=2^0
  pCANR_bool_MotCtlrTqVld : Inport  Port=3  OutDataType=fixdt(1, 16)  OutScaling=2^0
  bool_RcpTqLimBoostVld : Inport  Port=4  OutDataType=fixdt(1, 16)  OutScaling=2^0
  bool_DrvTqLimBoostVld : Inport  Port=5  OutDataType=fixdt(1, 16)  OutScaling=2^0
  pCANR_kmph_VehLgtSpd : Inport  Port=6  OutDataType=fixdt(1, 16)  OutScaling=2^0
  pCANR_rpm_MotCtlrActRev : Inport  Port=7  OutDataType=fixdt(1, 16)  OutScaling=2^0
  pCANR_Nm_MotCtlrActTq : Inport  Port=8  OutDataType=fixdt(1, 16)  OutScaling=2^0
  pCANR_Nm_RcpTqLimBoost : Inport  Port=9  OutDataType=fixdt(1, 16)  OutScaling=2^0
  pCANR_Nm_DrvTqLimBoost : Inport  Port=10  OutDataType=fixdt(1, 16)  OutScaling=2^0
  pCANR_st_CoolingRequest : Inport  Port=11  OutDataType=fixdt(1, 16)  OutScaling=2^0
  pCANR_Nm_CalTMTorque : Inport  Port=12  OutDataType=fixdt(1, 16)  OutScaling=2^0
  pCANR_bool_PrechargeAllow : Inport  Port=13  OutDataType=fixdt(1, 16)  OutScaling=2^0
  pCANR_V_MotCpU : Inport  Port=14  OutDataType=fixdt(1, 16)  OutScaling=2^0
  pCANR_st_TMStatus : Inport  Port=15  OutDataType=fixdt(1, 16)  OutScaling=2^0
  pCANR_st_MCU21TMErrSt : Inport  Port=16  OutDataType=fixdt(1, 16)  OutScaling=2^0
  pCANR_bool_MCU2ShtdwnAllow : Inport  Port=17  OutDataType=fixdt(1, 16)  OutScaling=2^0
  Constant : BaseOperationLib_Browser/Sources&Sinks/Constant  Value=pMCI_rpm_InsteadVld_C  OutMin=[]  OutMax=[]  OutDataTypeMode=single  OutDataType=fixdt(1, 16)  ConRadixGroup=Use specified scaling  OutScaling=2^0  OutDataTypeStr=single
  Constant1 : BaseOperationLib_Browser/Sources&Sinks/Constant  Value=uint8(MotCtrlWrkStsTyp.MCWS_TORQUE_CONTROL)  OutMin=[]  OutMax=[]  OutDataType=fixdt(1, 16)  ConRadixGroup=Use specified scaling  OutScaling=2^0  OutDataTypeStr=Inherit: Inherit from 'Constant value'
  Constant2 : BaseOperationLib_Browser/Sources&Sinks/Constant  Value=p_bool_False_M  OutMin=[]  OutMax=[]  OutDataType=fixdt(1, 16)  ConRadixGroup=Use specified scaling  OutScaling=2^0  OutDataTypeStr=Inherit: Inherit from 'Constant value'
  Constant5 : BaseOperationLib_Browser/Sources&Sinks/Constant  Value=p_bool_True_M  OutMin=[]  OutMax=[]  OutDataType=fixdt(1, 16)  ConRadixGroup=Use specified scaling  OutScaling=2^0  OutDataTypeStr=Inherit: Inherit from 'Constant value'
  Data Type Conversion{,1..4} (5 alike) : DataTypeConversion  OutDataType=fixdt(1, 16)  OutScaling=2^0
  Relational Operator : BaseOperationLib_Browser/Logic Operations Changed/Relational Operator  Operator=~=  InputSameDT=on  LogicOutDataTypeMode=Specify via dialog  LogicDataType=PDT_Bool  OutDataTypeStr=PDT_Bool
  Switch : BaseOperationLib_Browser/Signal Routing Changed/Switch  Criteria=u2 ~= 0  Threshold=1  InputSameDT=on  OutMin=[]  OutMax=[]  OutDataType=fixdt(1,16,0)  OutScaling=[]  SaturateOnIntegerOverflow=on
  Switch1 : BaseOperationLib_Browser/Signal Routing Changed/Switch  Criteria=u2 ~= 0  Threshold=1  InputSameDT=on  OutMin=[]  OutMax=[]  OutDataType=fixdt(1,16,0)  OutScaling=[]  SaturateOnIntegerOverflow=on
  Switch2 : BaseOperationLib_Browser/Signal Routing Changed/Switch  Criteria=u2 ~= 0  Threshold=1  InputSameDT=on  OutMin=[]  OutMax=[]  OutDataType=fixdt(1,16,0)  OutScaling=[]  SaturateOnIntegerOverflow=on
  Terminator : Terminator
  motor_efficiency_maps : Subsystem
  override : Subsystem
  override1 : Subsystem
  speed_to_rev : Subsystem
  valid_check3 : PES_CZ_FAW/Discontinuities/valid_check  SystemSampleTime=-1  init=0
  valid_check4 : PES_CZ_FAW/Discontinuities/valid_check  SystemSampleTime=-1  init=0
  valid_check5 : PES_CZ_FAW/Discontinuities/valid_check  SystemSampleTime=-1  init=0
  pMCI_rpm_MCU2MotCtrlActRev : Outport  OutDataType=fixdt(1, 16)  OutScaling=2^0
  pMCI_pct_MCU2MotDrvEffi : Outport  Port=2  OutDataType=fixdt(1, 16)  OutScaling=2^0
  pMCI_pct_MCU2MotRcpEffi : Outport  Port=3  OutDataType=fixdt(1, 16)  OutScaling=2^0
  pMCI_Nm_MCU2MotCtrlActTrq : Outport  Port=4  OutDataType=fixdt(1, 16)  OutScaling=2^0
  pMCI_Nm_MCU2RcpTrqLim : Outport  Port=5  OutDataType=fixdt(1, 16)  OutScaling=2^0
  pMCI_Nm_MCU2DrvTrqLim : Outport  Port=6  OutDataType=fixdt(1, 16)  OutScaling=2^0
  pMCI_st_MCU2CoolgReq : Outport  Port=7  OutDataType=fixdt(1, 16)  OutScaling=2^0
  pMCI_Nm_MCU2CalcTMTrq : Outport  Port=8  OutDataType=fixdt(1, 16)  OutScaling=2^0
  pMCI_bool_MCU2PreChrgAllow : Outport  Port=9  OutDataType=fixdt(1, 16)  OutScaling=2^0
  pMCI_V_MCU2MotCapVolt : Outport  Port=10  OutDataType=fixdt(1, 16)  OutScaling=2^0
  pMCI_st_MCU2MotCtrlWrkSt : Outport  Port=11  OutDataType=fixdt(1, 16)  OutScaling=2^0
  pMCI_bool_MCU2ShtdwnAllow : Outport  Port=12
  pMCI_bool_MCU2RpdDisChrgAllow : Outport  Port=13  OutDataType=fixdt(1, 16)  OutScaling=2^0
  wires:
  Data Type Conversion4/1 -> pMCI_st_MCU2CoolgReq/1
  Data Type Conversion3/1 -> pMCI_V_MCU2MotCapVolt/1
  Data Type Conversion2/1 -> pMCI_bool_MCU2PreChrgAllow/1
  Data Type Conversion/1 -> pMCI_Nm_MCU2CalcTMTrq/1
  pCANR_bool_PrechargeAllow/1 -> Data Type Conversion2/1
  pCANR_V_MotCpU/1 -> Data Type Conversion3/1
  pCANR_Nm_CalTMTorque/1 -> Data Type Conversion/1
  pCANR_st_CoolingRequest/1 -> Data Type Conversion4/1
  pCANR_st_TMStatus/1 -> Data Type Conversion1/1, Relational Operator/1
  Data Type Conversion1/1 -> pMCI_st_MCU2MotCtrlWrkSt/1
  override1/1(Out1) -> pMCI_Nm_MCU2DrvTrqLim/1
  override/1(Out1) -> pMCI_Nm_MCU2RcpTrqLim/1
  valid_check5/1 -> override1/1(In1)
  valid_check4/1 -> override/1(In1)
  pCANR_Nm_DrvTqLimBoost/1 -> valid_check5/1
  pCANR_Nm_RcpTqLimBoost/1 -> valid_check4/1
  bool_DrvTqLimBoostVld/1 -> valid_check5/2
  bool_RcpTqLimBoostVld/1 -> valid_check4/2
  valid_check3/1 -> pMCI_Nm_MCU2MotCtrlActTrq/1, motor_efficiency_maps/2(Nm_MotCtrlActTrq)
  pCANR_bool_MotCtlrTqVld/1 -> valid_check3/2
  pCANR_Nm_MotCtlrActTq/1 -> valid_check3/1
  motor_efficiency_maps/2(pct_MotRcpEffi) -> pMCI_pct_MCU2MotRcpEffi/1
  motor_efficiency_maps/1(pct_MotDrvEffi) -> pMCI_pct_MCU2MotDrvEffi/1
  Switch/1 -> Switch1/3
  pCANR_rpm_MotCtlrActRev/1 -> Switch1/1
  bool_MotCtlrActRevVld/1 -> Switch1/2
  pCANR_kmph_VehLgtSpd/1 -> speed_to_rev/1(VehLgtSpd_kmph)
  speed_to_rev/1(MotCtlrActRev_1pmin) -> Switch/1
  Constant/1 -> Switch/3
  bool_VehLgtSpdVld/1 -> Switch/2
  Switch1/1 -> motor_efficiency_maps/1(rpm_MotCtrlActRev), pMCI_rpm_MCU2MotCtrlActRev/1
  Constant5/1 -> pMCI_bool_MCU2RpdDisChrgAllow/1
  Constant1/1 -> Relational Operator/2
  pCANR_st_MCU21TMErrSt/1 -> Terminator/1
  pCANR_bool_MCU2ShtdwnAllow/1 -> Switch2/3
  Constant2/1 -> Switch2/2
  Relational Operator/1 -> Switch2/1
  Switch2/1 -> pMCI_bool_MCU2ShtdwnAllow/1

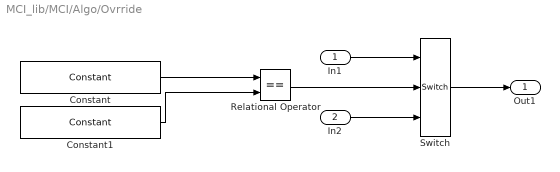
== system MCI_lib/MCI/Algo/Ovrride ==
  In1 : Inport  OutDataType=fixdt(1, 16)  OutScaling=2^0
  In2 : Inport  Port=2  OutDataType=fixdt(1, 16)  OutScaling=2^0
  Constant : BaseOperationLib_Browser/Sources&Sinks/Constant  Value=p_st_DrvModeFlg_C  OutMin=[]  OutMax=[]  OutDataType=fixdt(1, 16)  ConRadixGroup=Use specified scaling  OutScaling=2^0  OutDataTypeStr=Inherit: Inherit from 'Constant value'
  Constant1 : BaseOperationLib_Browser/Sources&Sinks/Constant  Value=1  OutMin=[]  OutMax=[]  OutDataTypeMode=uint8  OutDataType=fixdt(1, 16)  ConRadixGroup=Use specified scaling  OutScaling=2^0  OutDataTypeStr=uint8
  Relational Operator : RelationalOperator  Operator===  LogicOutDataTypeMode=boolean  LogicDataType=fixdt(0, 8)  OutDataTypeStr=boolean
  Switch : BaseOperationLib_Browser/Signal Routing Changed/Switch  Criteria=u2 ~= 0  Threshold=1  InputSameDT=on  OutMin=[]  OutMax=[]  OutDataType=fixdt(1,16,0)  OutScaling=[]  SaturateOnIntegerOverflow=on
  Out1 : Outport  OutDataType=fixdt(1, 16)  OutScaling=2^0
  wires:
  Relational Operator/1 -> Switch/2
  Switch/1 -> Out1/1
  In1/1 -> Switch/1
  In2/1 -> Switch/3
  Constant/1 -> Relational Operator/1
  Constant1/1 -> Relational Operator/2

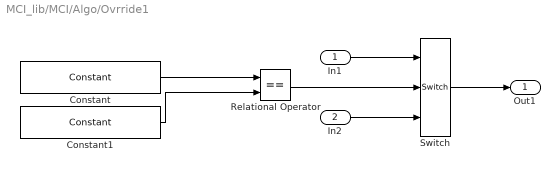
== system MCI_lib/MCI/Algo/Ovrride1 ==
  In1 : Inport  OutDataType=fixdt(1, 16)  OutScaling=2^0
  In2 : Inport  Port=2  OutDataType=fixdt(1, 16)  OutScaling=2^0
  Constant : BaseOperationLib_Browser/Sources&Sinks/Constant  Value=p_st_DrvModeFlg_C  OutMin=[]  OutMax=[]  OutDataType=fixdt(1, 16)  ConRadixGroup=Use specified scaling  OutScaling=2^0  OutDataTypeStr=Inherit: Inherit from 'Constant value'
  Constant1 : BaseOperationLib_Browser/Sources&Sinks/Constant  Value=1  OutMin=[]  OutMax=[]  OutDataTypeMode=uint8  OutDataType=fixdt(1, 16)  ConRadixGroup=Use specified scaling  OutScaling=2^0  OutDataTypeStr=uint8
  Relational Operator : RelationalOperator  Operator===  LogicOutDataTypeMode=boolean  LogicDataType=fixdt(0, 8)  OutDataTypeStr=boolean
  Switch : BaseOperationLib_Browser/Signal Routing Changed/Switch  Criteria=u2 ~= 0  Threshold=1  InputSameDT=on  OutMin=[]  OutMax=[]  OutDataType=fixdt(1,16,0)  OutScaling=[]  SaturateOnIntegerOverflow=on
  Out1 : Outport  OutDataType=fixdt(1, 16)  OutScaling=2^0
  wires:
  In2/1 -> Switch/3
  In1/1 -> Switch/1
  Switch/1 -> Out1/1
  Relational Operator/1 -> Switch/2
  Constant/1 -> Relational Operator/1
  Constant1/1 -> Relational Operator/2

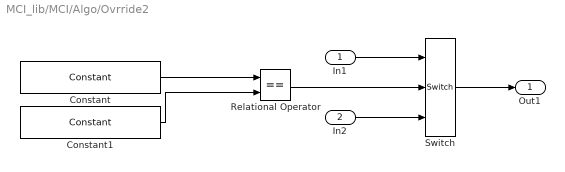
== system MCI_lib/MCI/Algo/Ovrride2 ==
  In1 : Inport  OutDataType=fixdt(1, 16)  OutScaling=2^0
  In2 : Inport  Port=2  OutDataType=fixdt(1, 16)  OutScaling=2^0
  Constant : BaseOperationLib_Browser/Sources&Sinks/Constant  Value=p_st_DrvModeFlg_C  OutMin=[]  OutMax=[]  OutDataType=fixdt(1, 16)  ConRadixGroup=Use specified scaling  OutScaling=2^0  OutDataTypeStr=Inherit: Inherit from 'Constant value'
  Constant1 : BaseOperationLib_Browser/Sources&Sinks/Constant  Value=1  OutMin=[]  OutMax=[]  OutDataTypeMode=uint8  OutDataType=fixdt(1, 16)  ConRadixGroup=Use specified scaling  OutScaling=2^0  OutDataTypeStr=uint8
  Relational Operator : RelationalOperator  Operator===  LogicOutDataTypeMode=boolean  LogicDataType=fixdt(0, 8)  OutDataTypeStr=boolean
  Switch : BaseOperationLib_Browser/Signal Routing Changed/Switch  Criteria=u2 ~= 0  Threshold=1  InputSameDT=on  OutMin=[]  OutMax=[]  OutDataType=fixdt(1,16,0)  OutScaling=[]  SaturateOnIntegerOverflow=on
  Out1 : Outport  OutDataType=fixdt(1, 16)  OutScaling=2^0
  wires:
  Relational Operator/1 -> Switch/2
  Switch/1 -> Out1/1
  In1/1 -> Switch/1
  In2/1 -> Switch/3
  Constant/1 -> Relational Operator/1
  Constant1/1 -> Relational Operator/2

== system MCI_lib/MCI/Algo/Ovrride3 ==
  In1 : Inport  OutDataType=fixdt(1, 16)  OutScaling=2^0
  In2 : Inport  Port=2  OutDataType=fixdt(1, 16)  OutScaling=2^0
  Constant : BaseOperationLib_Browser/Sources&Sinks/Constant  Value=p_st_DrvModeFlg_C  OutMin=[]  OutMax=[]  OutDataType=fixdt(1, 16)  ConRadixGroup=Use specified scaling  OutScaling=2^0  OutDataTypeStr=Inherit: Inherit from 'Constant value'
  Constant1 : BaseOperationLib_Browser/Sources&Sinks/Constant  Value=2  OutMin=[]  OutMax=[]  OutDataTypeMode=uint8  OutDataType=fixdt(1, 16)  ConRadixGroup=Use specified scaling  OutScaling=2^0  OutDataTypeStr=uint8
  Relational Operator : RelationalOperator  Operator=~=  LogicOutDataTypeMode=boolean  LogicDataType=fixdt(0, 8)  OutDataTypeStr=boolean
  Switch : BaseOperationLib_Browser/Signal Routing Changed/Switch  Criteria=u2 ~= 0  Threshold=1  InputSameDT=on  OutMin=[]  OutMax=[]  OutDataType=fixdt(1,16,0)  OutScaling=[]  SaturateOnIntegerOverflow=on
  Out1 : Outport  OutDataType=fixdt(1, 16)  OutScaling=2^0
  wires:
  Relational Operator/1 -> Switch/2
  Switch/1 -> Out1/1
  In1/1 -> Switch/1
  In2/1 -> Switch/3
  Constant/1 -> Relational Operator/1
  Constant1/1 -> Relational Operator/2

== system MCI_lib/MCI/Algo/Ovrride4 ==
  In1 : Inport  OutDataType=fixdt(1, 16)  OutScaling=2^0
  In2 : Inport  Port=2  OutDataType=fixdt(1, 16)  OutScaling=2^0
  Constant : BaseOperationLib_Browser/Sources&Sinks/Constant  Value=p_st_DrvModeFlg_C  OutMin=[]  OutMax=[]  OutDataType=fixdt(1, 16)  ConRadixGroup=Use specified scaling  OutScaling=2^0  OutDataTypeStr=Inherit: Inherit from 'Constant value'
  Constant1 : BaseOperationLib_Browser/Sources&Sinks/Constant  Value=2  OutMin=[]  OutMax=[]  OutDataTypeMode=uint8  OutDataType=fixdt(1, 16)  ConRadixGroup=Use specified scaling  OutScaling=2^0  OutDataTypeStr=uint8
  Relational Operator : RelationalOperator  Operator=~=  LogicOutDataTypeMode=boolean  LogicDataType=fixdt(0, 8)  OutDataTypeStr=boolean
  Switch : BaseOperationLib_Browser/Signal Routing Changed/Switch  Criteria=u2 ~= 0  Threshold=1  InputSameDT=on  OutMin=[]  OutMax=[]  OutDataType=fixdt(1,16,0)  OutScaling=[]  SaturateOnIntegerOverflow=on
  Out1 : Outport  OutDataType=fixdt(1, 16)  OutScaling=2^0
  wires:
  Switch/1 -> Out1/1
  In1/1 -> Switch/1
  In2/1 -> Switch/3
  Constant/1 -> Relational Operator/1
  Relational Operator/1 -> Switch/2
  Constant1/1 -> Relational Operator/2

== system MCI_lib/MCI/Algo/Ovrride5 ==
  In1 : Inport  OutDataType=fixdt(1, 16)  OutScaling=2^0
  In2 : Inport  Port=2  OutDataType=fixdt(1, 16)  OutScaling=2^0
  Constant : BaseOperationLib_Browser/Sources&Sinks/Constant  Value=p_st_DrvModeFlg_C  OutMin=[]  OutMax=[]  OutDataType=fixdt(1, 16)  ConRadixGroup=Use specified scaling  OutScaling=2^0  OutDataTypeStr=Inherit: Inherit from 'Constant value'
  Constant1 : BaseOperationLib_Browser/Sources&Sinks/Constant  Value=2  OutMin=[]  OutMax=[]  OutDataTypeMode=uint8  OutDataType=fixdt(1, 16)  ConRadixGroup=Use specified scaling  OutScaling=2^0  OutDataTypeStr=uint8
  Relational Operator : RelationalOperator  Operator=~=  LogicOutDataTypeMode=boolean  LogicDataType=fixdt(0, 8)  OutDataTypeStr=boolean
  Switch : BaseOperationLib_Browser/Signal Routing Changed/Switch  Criteria=u2 ~= 0  Threshold=1  InputSameDT=on  OutMin=[]  OutMax=[]  OutDataType=fixdt(1,16,0)  OutScaling=[]  SaturateOnIntegerOverflow=on
  Out1 : Outport  OutDataType=fixdt(1, 16)  OutScaling=2^0
  wires:
  Relational Operator/1 -> Switch/2
  Switch/1 -> Out1/1
  In1/1 -> Switch/1
  In2/1 -> Switch/3
  Constant/1 -> Relational Operator/1
  Constant1/1 -> Relational Operator/2

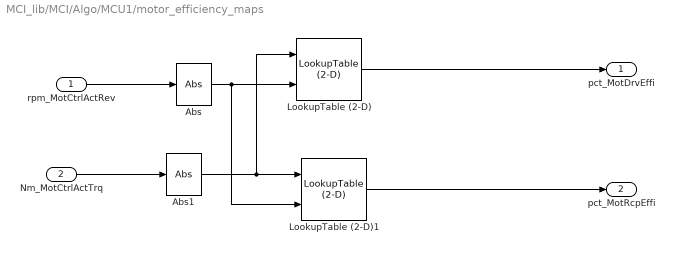
== system MCI_lib/MCI/Algo/MCU1/motor_efficiency_maps ==
  rpm_MotCtrlActRev : Inport  OutDataType=fixdt(1, 16)  OutScaling=2^0
  Nm_MotCtrlActTrq : Inport  Port=2  OutDataType=fixdt(1, 16)  OutScaling=2^0
  Abs : BaseOperationLib_Browser/Math Operations Changed/Abs  OutMax=[]  OutDataType=fixdt(1, 16)  OutScaling=2^0  SaturateOnIntegerOverflow=on
  Abs1 : BaseOperationLib_Browser/Math Operations Changed/Abs  OutMax=[]  OutDataType=fixdt(1, 16)  OutScaling=2^0  SaturateOnIntegerOverflow=on
  LookupTable (2-D) : BaseOperationLib_Browser/Lookup Tables Changed/LookupTable (2-D)  RowIndex=pMCI_Nm_DrvEffXTrq_TABX  ColumnIndex=pMCI_rpm_DrvEffXSpd_TABY  Table=pMCI_ratio_DrvEff_MAP  LookUpMeth=Interpolation-Use End Values  OutMin=[]  OutMax=[]  OutDataType=fixdt(1, 16)  OutScaling=2^0  OutDataTypeStr=Inherit: Inherit via back propagation  SaturateOnIntegerOverflow=on
      settings: AttributesFormatString=X:%<RowIndex>\nY:%<ColumnIndex>\nTAB:%<Table>
  LookupTable (2-D)1 : BaseOperationLib_Browser/Lookup Tables Changed/LookupTable (2-D)  RowIndex=pMCI_Nm_DrvEffXTrq_TABX  ColumnIndex=pMCI_rpm_DrvEffXSpd_TABY  Table=pMCI_ratio_DrvEff_MAP  LookUpMeth=Interpolation-Use End Values  OutMin=[]  OutMax=[]  OutDataType=fixdt(1, 16)  OutScaling=2^0  OutDataTypeStr=Inherit: Inherit via back propagation  SaturateOnIntegerOverflow=on
      settings: AttributesFormatString=X:%<RowIndex>\nY:%<ColumnIndex>\nTAB:%<Table>
  pct_MotDrvEffi : Outport
  pct_MotRcpEffi : Outport  Port=2
  wires:
  LookupTable (2-D)1/1 -> pct_MotRcpEffi/1
  Abs1/1 -> LookupTable (2-D)1/1, LookupTable (2-D)/1
  LookupTable (2-D)/1 -> pct_MotDrvEffi/1
  Nm_MotCtrlActTrq/1 -> Abs1/1
  rpm_MotCtrlActRev/1 -> Abs/1
  Abs/1 -> LookupTable (2-D)1/2, LookupTable (2-D)/2

== system MCI_lib/MCI/Algo/MCU1/override ==
  In1 : Inport
  ASR_switch : BaseOperationLib_Browser/Sources&Sinks/Constant  Value=pMCI_bool_MotCtrlTqLimEna_C  OutMin=[]  OutMax=[]  OutDataTypeMode=boolean  OutDataType=fixdt(1, 16)  ConRadixGroup=Use specified scaling  OutScaling=2^0  OutDataTypeStr=boolean
  Constant : BaseOperationLib_Browser/Sources&Sinks/Constant  Value=pMCI_Nm_RcpTqLim_C  OutMin=[]  OutMax=[]  OutDataTypeMode=single  OutDataType=fixdt(1, 16)  ConRadixGroup=Use specified scaling  OutScaling=2^0  OutDataTypeStr=single
  Switch1 : BaseOperationLib_Browser/Signal Routing Changed/Switch  Criteria=u2 ~= 0  Threshold=1  InputSameDT=on  OutMin=[]  OutMax=[]  OutDataType=fixdt(1,16,0)  OutScaling=[]  SaturateOnIntegerOverflow=on
  Out1 : Outport
  wires:
  Switch1/1 -> Out1/1
  In1/1 -> Switch1/1
  Constant/1 -> Switch1/3
  ASR_switch/1 -> Switch1/2

== system MCI_lib/MCI/Algo/MCU1/override1 ==
  In1 : Inport
  ASR_switch1 : BaseOperationLib_Browser/Sources&Sinks/Constant  Value=pMCI_bool_MotCtrlTqLimEna_C  OutMin=[]  OutMax=[]  OutDataTypeMode=boolean  OutDataType=fixdt(1, 16)  ConRadixGroup=Use specified scaling  OutScaling=2^0  OutDataTypeStr=boolean
  Constant1 : BaseOperationLib_Browser/Sources&Sinks/Constant  Value=pMCI_Nm_DrvTqLim_C  OutMin=[]  OutMax=[]  OutDataTypeMode=single  OutDataType=fixdt(1, 16)  ConRadixGroup=Use specified scaling  OutScaling=2^0  OutDataTypeStr=single
  Switch2 : BaseOperationLib_Browser/Signal Routing Changed/Switch  Criteria=u2 ~= 0  Threshold=1  InputSameDT=on  OutMin=[]  OutMax=[]  OutDataType=fixdt(1,16,0)  OutScaling=[]  SaturateOnIntegerOverflow=on
  Out1 : Outport
  wires:
  Switch2/1 -> Out1/1
  In1/1 -> Switch2/1
  Constant1/1 -> Switch2/3
  ASR_switch1/1 -> Switch2/2

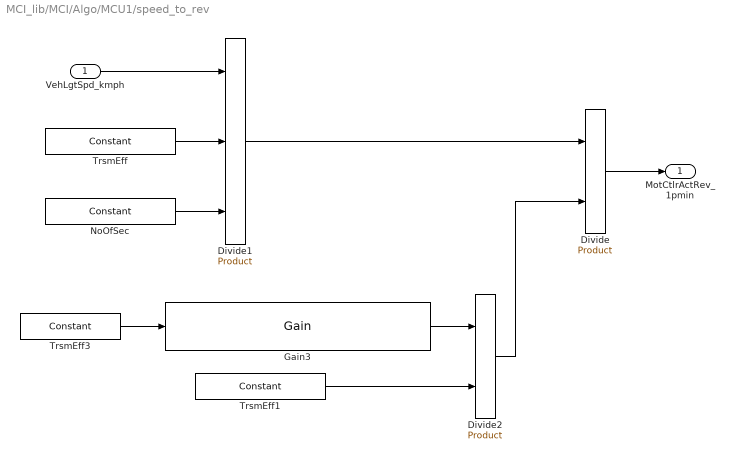
== system MCI_lib/MCI/Algo/MCU1/speed_to_rev ==
  VehLgtSpd_kmph : Inport
  Divide : BaseOperationLib_Browser/Math Operations Changed/Product  Inputs=*/  Multiplication=Element-wise(.*)  OutMin=[]  OutMax=[]  OutDataType=fixdt(1,16,0)  OutScaling=[]
  Divide1 : BaseOperationLib_Browser/Math Operations Changed/Product  Inputs=***  Multiplication=Element-wise(.*)  OutMin=[]  OutMax=[]  OutDataType=fixdt(1,16,0)  OutScaling=[]
  Divide2 : BaseOperationLib_Browser/Math Operations Changed/Product  Inputs=**  Multiplication=Element-wise(.*)  OutMin=[]  OutMax=[]  OutDataType=fixdt(1,16,0)  OutScaling=[]
  Gain3 : BaseOperationLib_Browser/Math Operations Changed/Gain  Gain=pMCI_ratio_KmPerHrToMtrPerSec_C  Multiplication=Element-wise(K.*u)  ParamMin=[]  ParamMax=[]  ParameterDataType=fixdt(1, 16)  ParameterScalingMode=Best Precision: Matrix-wise  ParameterScaling=2^0  OutMin=[]  OutMax=[]  OutDataType=fixdt(1, 16)  OutScaling=2^0
  NoOfSec : BaseOperationLib_Browser/Sources&Sinks/Constant  Value=pMCI_s_NoOfSec_C  OutMin=[]  OutMax=[]  OutDataTypeMode=single  OutDataType=fixdt(1, 16)  ConRadixGroup=Use specified scaling  OutScaling=2^0  OutDataTypeStr=single
  TrsmEff : BaseOperationLib_Browser/Sources&Sinks/Constant  Value=pMCI_ratio_TrsmRat_C  OutMin=[]  OutMax=[]  OutDataTypeMode=single  OutDataType=fixdt(1, 16)  ConRadixGroup=Use specified scaling  OutScaling=2^0  OutDataTypeStr=single
  TrsmEff1 : BaseOperationLib_Browser/Sources&Sinks/Constant  Value=pMCI_m_TireDiam_C  OutMin=[]  OutMax=[]  OutDataTypeMode=single  OutDataType=fixdt(1, 16)  ConRadixGroup=Use specified scaling  OutScaling=2^0  OutDataTypeStr=single
  TrsmEff3 : BaseOperationLib_Browser/Sources&Sinks/Constant  Value=pi  OutMin=[]  OutMax=[]  OutDataTypeMode=single  OutDataType=fixdt(1, 16)  ConRadixGroup=Use specified scaling  OutScaling=2^0  OutDataTypeStr=single
  MotCtlrActRev_1pmin : Outport
  wires:
  Divide2/1 -> Divide/2
  Divide1/1 -> Divide/1
  Gain3/1 -> Divide2/1
  TrsmEff3/1 -> Gain3/1
  NoOfSec/1 -> Divide1/3
  TrsmEff/1 -> Divide1/2
  VehLgtSpd_kmph/1 -> Divide1/1
  Divide/1 -> MotCtlrActRev_1pmin/1
  TrsmEff1/1 -> Divide2/2

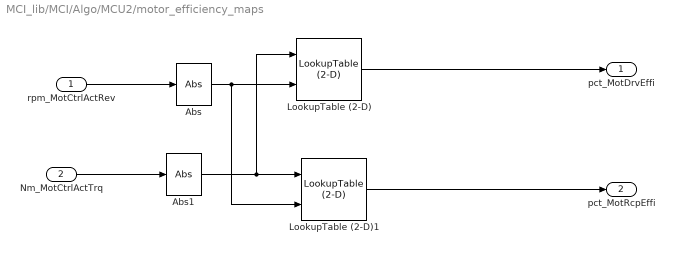
== system MCI_lib/MCI/Algo/MCU2/motor_efficiency_maps ==
  rpm_MotCtrlActRev : Inport  OutDataType=fixdt(1, 16)  OutScaling=2^0
  Nm_MotCtrlActTrq : Inport  Port=2  OutDataType=fixdt(1, 16)  OutScaling=2^0
  Abs : BaseOperationLib_Browser/Math Operations Changed/Abs  OutMax=[]  OutDataType=fixdt(1, 16)  OutScaling=2^0  SaturateOnIntegerOverflow=on
  Abs1 : BaseOperationLib_Browser/Math Operations Changed/Abs  OutMax=[]  OutDataType=fixdt(1, 16)  OutScaling=2^0  SaturateOnIntegerOverflow=on
  LookupTable (2-D) : BaseOperationLib_Browser/Lookup Tables Changed/LookupTable (2-D)  RowIndex=pMCI_Nm_DrvEffXTrq_TABX  ColumnIndex=pMCI_rpm_DrvEffXSpd_TABY  Table=pMCI_ratio_DrvEff_MAP  LookUpMeth=Interpolation-Use End Values  OutMin=[]  OutMax=[]  OutDataType=fixdt(1, 16)  OutScaling=2^0  OutDataTypeStr=Inherit: Inherit via back propagation  SaturateOnIntegerOverflow=on
      settings: AttributesFormatString=X:%<RowIndex>\nY:%<ColumnIndex>\nTAB:%<Table>
  LookupTable (2-D)1 : BaseOperationLib_Browser/Lookup Tables Changed/LookupTable (2-D)  RowIndex=pMCI_Nm_DrvEffXTrq_TABX  ColumnIndex=pMCI_rpm_DrvEffXSpd_TABY  Table=pMCI_ratio_DrvEff_MAP  LookUpMeth=Interpolation-Use End Values  OutMin=[]  OutMax=[]  OutDataType=fixdt(1, 16)  OutScaling=2^0  OutDataTypeStr=Inherit: Inherit via back propagation  SaturateOnIntegerOverflow=on
      settings: AttributesFormatString=X:%<RowIndex>\nY:%<ColumnIndex>\nTAB:%<Table>
  pct_MotDrvEffi : Outport
  pct_MotRcpEffi : Outport  Port=2
  wires:
  Abs/1 -> LookupTable (2-D)/2, LookupTable (2-D)1/2
  rpm_MotCtrlActRev/1 -> Abs/1
  Nm_MotCtrlActTrq/1 -> Abs1/1
  LookupTable (2-D)/1 -> pct_MotDrvEffi/1
  Abs1/1 -> LookupTable (2-D)/1, LookupTable (2-D)1/1
  LookupTable (2-D)1/1 -> pct_MotRcpEffi/1

== system MCI_lib/MCI/Algo/MCU2/override ==
  In1 : Inport
  ASR_switch : BaseOperationLib_Browser/Sources&Sinks/Constant  Value=pMCI_bool_MotCtrlTqLimEna_C  OutMin=[]  OutMax=[]  OutDataTypeMode=boolean  OutDataType=fixdt(1, 16)  ConRadixGroup=Use specified scaling  OutScaling=2^0  OutDataTypeStr=boolean
  Constant : BaseOperationLib_Browser/Sources&Sinks/Constant  Value=pMCI_Nm_RcpTqLim_C  OutMin=[]  OutMax=[]  OutDataTypeMode=single  OutDataType=fixdt(1, 16)  ConRadixGroup=Use specified scaling  OutScaling=2^0  OutDataTypeStr=single
  Switch1 : BaseOperationLib_Browser/Signal Routing Changed/Switch  Criteria=u2 ~= 0  Threshold=1  InputSameDT=on  OutMin=[]  OutMax=[]  OutDataType=fixdt(1,16,0)  OutScaling=[]  SaturateOnIntegerOverflow=on
  Out1 : Outport
  wires:
  ASR_switch/1 -> Switch1/2
  Constant/1 -> Switch1/3
  In1/1 -> Switch1/1
  Switch1/1 -> Out1/1

== system MCI_lib/MCI/Algo/MCU2/override1 ==
  In1 : Inport
  ASR_switch1 : BaseOperationLib_Browser/Sources&Sinks/Constant  Value=pMCI_bool_MotCtrlTqLimEna_C  OutMin=[]  OutMax=[]  OutDataTypeMode=boolean  OutDataType=fixdt(1, 16)  ConRadixGroup=Use specified scaling  OutScaling=2^0  OutDataTypeStr=boolean
  Constant1 : BaseOperationLib_Browser/Sources&Sinks/Constant  Value=pMCI_Nm_DrvTqLim_C  OutMin=[]  OutMax=[]  OutDataTypeMode=single  OutDataType=fixdt(1, 16)  ConRadixGroup=Use specified scaling  OutScaling=2^0  OutDataTypeStr=single
  Switch2 : BaseOperationLib_Browser/Signal Routing Changed/Switch  Criteria=u2 ~= 0  Threshold=1  InputSameDT=on  OutMin=[]  OutMax=[]  OutDataType=fixdt(1,16,0)  OutScaling=[]  SaturateOnIntegerOverflow=on
  Out1 : Outport
  wires:
  ASR_switch1/1 -> Switch2/2
  Constant1/1 -> Switch2/3
  In1/1 -> Switch2/1
  Switch2/1 -> Out1/1
